simulink model "dog_x_bit_true_2024"  (R2024a)
settings: Solver=ode45  StartTime=0.0  StopTime=1.5*lsim*Ts  MaxStep=1/f0/2  RelTol=1e-6
values from neighbouring files (symbols this model uses):
  ft = (bint-1)*fbin    [exe_DOG_X_bit_true_2023a.m]    (also in exe_DOG_X_integer_true_two_paths_5b.m)
  g1 = g1_ideal*1    (= 4)    [exe_DOG_X_bit_true_2023a.m]    (also in exe_DOG_X_integer_true_two_paths_5b.m)
  Kvco = f0    (= 99840000)    [exe_DOG_X_bit_true_2023a.m]    (also in exe_DOG_X_integer_true_two_paths_5b.m)
  lvl = Vfs*10^(Input_signal_dB/20)    (= 0.125892541179)    [exe_DOG_X_bit_true_2023a.m]    (also in exe_DOG_X_integer_true_two_paths_5b.m)
  Nbsv1 = Nbvco+4    (= 9)    [exe_DOG_X_bit_true_2023a.m]    (also in exe_DOG_X_integer_true_two_paths_5b.m)
  Nbsv2 = Nbsv1+Nbext    [exe_DOG_X_bit_true_2023a.m]    (also in exe_DOG_X_integer_true_two_paths_5b.m)
  pnoi = 10^(-(60)/10)*(Vfs^2/2)    (= 5e-07)    [exe_DOG_X_bit_true_2023a.m]    (also in exe_DOG_X_integer_true_two_paths_5b.m)
  T2 = 1/f2    (= 4.06901041667e-08)    [exe_DOG_X_bit_true_2023a.m]    (also in exe_DOG_X_integer_true_two_paths_5b.m)
  Ts = 1/fs    (= 3.25520833333e-07)    [exe_DOG_X_bit_true_2023a.m]    (also in exe_DOG_X_integer_true_two_paths_5b.m)
  Vfs = 1    [exe_DOG_X_bit_true_2023a.m]    (also in exe_DOG_X_integer_true_two_paths_5b.m)
undefined symbols (not defined in the file or in its folder): fa, fb
libraries: simulink_extras x86, simulink x8
(part 3 of 4)

== system dog_x_bit_true_2024/TOP/Subsystem/progressive_mux/Subsystem1 ==
  select : Inport
  A : Inport  Port=2
  B : Inport  Port=3
  AND : Logic  IconShape=distinctive  AllPortsSameDT=off  OutDataTypeStr=boolean
  AND1 : Logic  IconShape=distinctive  AllPortsSameDT=off  OutDataTypeStr=boolean
  Demux : Demux  Outputs=15
  FA1 : Subsystem
  FA10 : Subsystem
  FA11 : Subsystem
  FA2 : Subsystem
  FA3 : Subsystem
  FA4 : Subsystem
  FA5 : Subsystem
  FA6 : Subsystem
  FA7 : Subsystem
  FA8 : Subsystem
  FA9 : Subsystem
  Mux : Mux
  NOT : Logic  Operator=NOT  IconShape=distinctive  AllPortsSameDT=off  OutDataTypeStr=boolean
  OR : Logic  Operator=OR  IconShape=distinctive  AllPortsSameDT=off  OutDataTypeStr=boolean
  Y : Outport
  wires:
  AND/1 -> OR/1
  A/1 -> AND/1
  AND1/1 -> OR/2
  B/1 -> AND1/2
  select/1 -> NOT/1, AND/2
  NOT/1 -> AND1/1
  OR/1 -> Demux/1
  Demux/2 -> FA10/3(Cin)
  Demux/15 -> FA10/1(B0)
  Demux/14 -> FA1/3(Cin)
  Demux/13 -> FA1/2(B1)
  Demux/12 -> FA1/1(B0)
  FA1/1(S) -> FA4/1(B0)
  FA10/1(S) -> FA4/2(B1)
  FA1/2(Co) -> FA5/2(B1)
  FA10/2(Co) -> FA5/1(B0)
  FA4/2(Co) -> FA5/3(Cin)
  Demux/11 -> FA4/3(Cin)
  FA6/2(Co) -> FA7/3(Cin)
  Demux/4 -> FA6/3(Cin)
  FA3/2(Co) -> FA7/1(B0)
  Demux/7 -> FA2/3(Cin)
  Demux/10 -> FA3/3(Cin)
  FA2/2(Co) -> FA7/2(B1)
  Demux/6 -> FA2/2(B1)
  Demux/9 -> FA3/2(B1)
  FA2/1(S) -> FA6/1(B0)
  FA3/1(S) -> FA6/2(B1)
  Demux/8 -> FA3/1(B0)
  Demux/5 -> FA2/1(B0)
  FA4/1(S) -> FA8/2(B1)
  FA5/1(S) -> FA9/2(B1)
  FA5/2(Co) -> FA11/2(B1)
  FA6/1(S) -> FA8/1(B0)
  FA7/1(S) -> FA9/1(B0)
  FA7/2(Co) -> FA11/1(B0)
  Demux/3 -> FA8/3(Cin)
  FA8/2(Co) -> FA9/3(Cin)
  FA9/2(Co) -> FA11/3(Cin)
  Demux/1 -> FA10/2(B1)
  FA11/2(Co) -> Mux/1
  FA11/1(S) -> Mux/2
  FA9/1(S) -> Mux/3
  FA8/1(S) -> Mux/4
  Mux/1 -> Y/1

== system dog_x_bit_true_2024/TOP/alpha2/abs/FA10 ==
  B0 : Inport
  B1 : Inport  Port=2
  Cin : Inport  Port=3
  Combinatorial Logic : CombinatorialLogic
  Demux : Demux  Outputs=2
  Mux : Mux  Inputs=3
  S : Outport
  Co : Outport  Port=2
  wires:
  Mux/1 -> Combinatorial Logic/1
  Combinatorial Logic/1 -> Demux/1
  B1/1 -> Mux/2
  Cin/1 -> Mux/3
  B0/1 -> Mux/1
  Demux/1 -> Co/1
  Demux/2 -> S/1

== system dog_x_bit_true_2024/TOP/alpha2/abs/FA2 ==
  B0 : Inport
  B1 : Inport  Port=2
  Cin : Inport  Port=3
  Combinatorial Logic : CombinatorialLogic
  Demux : Demux  Outputs=2
  Mux : Mux  Inputs=3
  S : Outport
  Co : Outport  Port=2
  wires:
  Mux/1 -> Combinatorial Logic/1
  Combinatorial Logic/1 -> Demux/1
  B1/1 -> Mux/2
  Cin/1 -> Mux/3
  B0/1 -> Mux/1
  Demux/1 -> Co/1
  Demux/2 -> S/1

== system dog_x_bit_true_2024/TOP/alpha2/abs/FA3 ==
  B0 : Inport
  B1 : Inport  Port=2
  Cin : Inport  Port=3
  Combinatorial Logic : CombinatorialLogic
  Demux : Demux  Outputs=2
  Mux : Mux  Inputs=3
  S : Outport
  Co : Outport  Port=2
  wires:
  Mux/1 -> Combinatorial Logic/1
  Combinatorial Logic/1 -> Demux/1
  B1/1 -> Mux/2
  Cin/1 -> Mux/3
  B0/1 -> Mux/1
  Demux/1 -> Co/1
  Demux/2 -> S/1

== system dog_x_bit_true_2024/TOP/alpha2/abs/FA4 ==
  B0 : Inport
  B1 : Inport  Port=2
  Cin : Inport  Port=3
  Combinatorial Logic : CombinatorialLogic
  Demux : Demux  Outputs=2
  Mux : Mux  Inputs=3
  S : Outport
  Co : Outport  Port=2
  wires:
  Mux/1 -> Combinatorial Logic/1
  Combinatorial Logic/1 -> Demux/1
  B1/1 -> Mux/2
  Cin/1 -> Mux/3
  B0/1 -> Mux/1
  Demux/1 -> Co/1
  Demux/2 -> S/1

== system dog_x_bit_true_2024/TOP/alpha2/abs/FA5 ==
  B0 : Inport
  B1 : Inport  Port=2
  Cin : Inport  Port=3
  Combinatorial Logic : CombinatorialLogic
  Demux : Demux  Outputs=2
  Mux : Mux  Inputs=3
  S : Outport
  Co : Outport  Port=2
  wires:
  Mux/1 -> Combinatorial Logic/1
  Combinatorial Logic/1 -> Demux/1
  B1/1 -> Mux/2
  Cin/1 -> Mux/3
  B0/1 -> Mux/1
  Demux/1 -> Co/1
  Demux/2 -> S/1

== system dog_x_bit_true_2024/TOP/alpha2/abs/FA6 ==
  B0 : Inport
  B1 : Inport  Port=2
  Cin : Inport  Port=3
  Combinatorial Logic : CombinatorialLogic
  Demux : Demux  Outputs=2
  Mux : Mux  Inputs=3
  S : Outport
  Co : Outport  Port=2
  wires:
  Mux/1 -> Combinatorial Logic/1
  Combinatorial Logic/1 -> Demux/1
  B1/1 -> Mux/2
  Cin/1 -> Mux/3
  B0/1 -> Mux/1
  Demux/1 -> Co/1
  Demux/2 -> S/1

== system dog_x_bit_true_2024/TOP/alpha2/abs/FA7 ==
  B0 : Inport
  B1 : Inport  Port=2
  Cin : Inport  Port=3
  Combinatorial Logic : CombinatorialLogic
  Demux : Demux  Outputs=2
  Mux : Mux  Inputs=3
  S : Outport
  Co : Outport  Port=2
  wires:
  Mux/1 -> Combinatorial Logic/1
  Combinatorial Logic/1 -> Demux/1
  B1/1 -> Mux/2
  Cin/1 -> Mux/3
  B0/1 -> Mux/1
  Demux/1 -> Co/1
  Demux/2 -> S/1

== system dog_x_bit_true_2024/TOP/alpha2/abs/FA9 ==
  B0 : Inport
  Cin : Inport  Port=2
  B1 : Inport  Port=3
  Combinatorial Logic : CombinatorialLogic
  Demux : Demux  Outputs=2
  Mux : Mux  Inputs=3
  S : Outport
  Co : Outport  Port=2
  wires:
  Mux/1 -> Combinatorial Logic/1
  Combinatorial Logic/1 -> Demux/1
  B1/1 -> Mux/2
  Cin/1 -> Mux/3
  B0/1 -> Mux/1
  Demux/1 -> Co/1
  Demux/2 -> S/1

== system dog_x_bit_true_2024/TOP/alpha2/comp_HI_Threshold/FA1 ==
  B0 : Inport
  B1 : Inport  Port=2
  Cin : Inport  Port=3
  Combinatorial Logic : CombinatorialLogic
  Demux : Demux  Outputs=2
  Mux : Mux  Inputs=3
  S : Outport
  Co : Outport  Port=2
  wires:
  Mux/1 -> Combinatorial Logic/1
  Combinatorial Logic/1 -> Demux/1
  B1/1 -> Mux/2
  Cin/1 -> Mux/3
  B0/1 -> Mux/1
  Demux/1 -> Co/1
  Demux/2 -> S/1

== system dog_x_bit_true_2024/TOP/alpha2/comp_HI_Threshold/FA10 ==
  B0 : Inport
  B1 : Inport  Port=2
  Cin : Inport  Port=3
  Combinatorial Logic : CombinatorialLogic
  Demux : Demux  Outputs=2
  Mux : Mux  Inputs=3
  S : Outport
  Co : Outport  Port=2
  wires:
  Mux/1 -> Combinatorial Logic/1
  Combinatorial Logic/1 -> Demux/1
  B1/1 -> Mux/2
  Cin/1 -> Mux/3
  B0/1 -> Mux/1
  Demux/1 -> Co/1
  Demux/2 -> S/1

== system dog_x_bit_true_2024/TOP/alpha2/comp_HI_Threshold/FA2 ==
  B0 : Inport
  B1 : Inport  Port=2
  Cin : Inport  Port=3
  Combinatorial Logic : CombinatorialLogic
  Demux : Demux  Outputs=2
  Mux : Mux  Inputs=3
  S : Outport
  Co : Outport  Port=2
  wires:
  Mux/1 -> Combinatorial Logic/1
  Combinatorial Logic/1 -> Demux/1
  B1/1 -> Mux/2
  Cin/1 -> Mux/3
  B0/1 -> Mux/1
  Demux/1 -> Co/1
  Demux/2 -> S/1

== system dog_x_bit_true_2024/TOP/alpha2/comp_HI_Threshold/FA3 ==
  B0 : Inport
  B1 : Inport  Port=2
  Cin : Inport  Port=3
  Combinatorial Logic : CombinatorialLogic
  Demux : Demux  Outputs=2
  Mux : Mux  Inputs=3
  S : Outport
  Co : Outport  Port=2
  wires:
  Mux/1 -> Combinatorial Logic/1
  Combinatorial Logic/1 -> Demux/1
  B1/1 -> Mux/2
  Cin/1 -> Mux/3
  B0/1 -> Mux/1
  Demux/1 -> Co/1
  Demux/2 -> S/1

== system dog_x_bit_true_2024/TOP/alpha2/comp_HI_Threshold/FA4 ==
  B0 : Inport
  B1 : Inport  Port=2
  Cin : Inport  Port=3
  Combinatorial Logic : CombinatorialLogic
  Demux : Demux  Outputs=2
  Mux : Mux  Inputs=3
  S : Outport
  Co : Outport  Port=2
  wires:
  Mux/1 -> Combinatorial Logic/1
  Combinatorial Logic/1 -> Demux/1
  B1/1 -> Mux/2
  Cin/1 -> Mux/3
  B0/1 -> Mux/1
  Demux/1 -> Co/1
  Demux/2 -> S/1

== system dog_x_bit_true_2024/TOP/alpha2/comp_HI_Threshold/FA5 ==
  B0 : Inport
  B1 : Inport  Port=2
  Cin : Inport  Port=3
  Combinatorial Logic : CombinatorialLogic
  Demux : Demux  Outputs=2
  Mux : Mux  Inputs=3
  S : Outport
  Co : Outport  Port=2
  wires:
  Mux/1 -> Combinatorial Logic/1
  Combinatorial Logic/1 -> Demux/1
  B1/1 -> Mux/2
  Cin/1 -> Mux/3
  B0/1 -> Mux/1
  Demux/1 -> Co/1
  Demux/2 -> S/1

== system dog_x_bit_true_2024/TOP/alpha2/comp_HI_Threshold/FA6 ==
  B0 : Inport
  B1 : Inport  Port=2
  Cin : Inport  Port=3
  Combinatorial Logic : CombinatorialLogic
  Demux : Demux  Outputs=2
  Mux : Mux  Inputs=3
  S : Outport
  Co : Outport  Port=2
  wires:
  Mux/1 -> Combinatorial Logic/1
  Combinatorial Logic/1 -> Demux/1
  B1/1 -> Mux/2
  Cin/1 -> Mux/3
  B0/1 -> Mux/1
  Demux/1 -> Co/1
  Demux/2 -> S/1

== system dog_x_bit_true_2024/TOP/alpha2/comp_HI_Threshold/FA7 ==
  B0 : Inport
  B1 : Inport  Port=2
  Cin : Inport  Port=3
  Combinatorial Logic : CombinatorialLogic
  Demux : Demux  Outputs=2
  Mux : Mux  Inputs=3
  S : Outport
  Co : Outport  Port=2
  wires:
  Mux/1 -> Combinatorial Logic/1
  Combinatorial Logic/1 -> Demux/1
  B1/1 -> Mux/2
  Cin/1 -> Mux/3
  B0/1 -> Mux/1
  Demux/1 -> Co/1
  Demux/2 -> S/1

== system dog_x_bit_true_2024/TOP/alpha2/comp_HI_Threshold/FA9 ==
  B0 : Inport
  Cin : Inport  Port=2
  B1 : Inport  Port=3
  Combinatorial Logic : CombinatorialLogic
  Demux : Demux  Outputs=2
  Mux : Mux  Inputs=3
  S : Outport
  Co : Outport  Port=2
  wires:
  Mux/1 -> Combinatorial Logic/1
  Combinatorial Logic/1 -> Demux/1
  B1/1 -> Mux/2
  Cin/1 -> Mux/3
  B0/1 -> Mux/1
  Demux/1 -> Co/1
  Demux/2 -> S/1

== system dog_x_bit_true_2024/TOP/alpha2/comp_LOW_Threshold/FA1 ==
  B0 : Inport
  B1 : Inport  Port=2
  Cin : Inport  Port=3
  Combinatorial Logic : CombinatorialLogic
  Demux : Demux  Outputs=2
  Mux : Mux  Inputs=3
  S : Outport
  Co : Outport  Port=2
  wires:
  Mux/1 -> Combinatorial Logic/1
  Combinatorial Logic/1 -> Demux/1
  B1/1 -> Mux/2
  Cin/1 -> Mux/3
  B0/1 -> Mux/1
  Demux/1 -> Co/1
  Demux/2 -> S/1

== system dog_x_bit_true_2024/TOP/alpha2/comp_LOW_Threshold/FA10 ==
  B0 : Inport
  B1 : Inport  Port=2
  Cin : Inport  Port=3
  Combinatorial Logic : CombinatorialLogic
  Demux : Demux  Outputs=2
  Mux : Mux  Inputs=3
  S : Outport
  Co : Outport  Port=2
  wires:
  Mux/1 -> Combinatorial Logic/1
  Combinatorial Logic/1 -> Demux/1
  B1/1 -> Mux/2
  Cin/1 -> Mux/3
  B0/1 -> Mux/1
  Demux/1 -> Co/1
  Demux/2 -> S/1

== system dog_x_bit_true_2024/TOP/alpha2/comp_LOW_Threshold/FA2 ==
  B0 : Inport
  B1 : Inport  Port=2
  Cin : Inport  Port=3
  Combinatorial Logic : CombinatorialLogic
  Demux : Demux  Outputs=2
  Mux : Mux  Inputs=3
  S : Outport
  Co : Outport  Port=2
  wires:
  Mux/1 -> Combinatorial Logic/1
  Combinatorial Logic/1 -> Demux/1
  B1/1 -> Mux/2
  Cin/1 -> Mux/3
  B0/1 -> Mux/1
  Demux/1 -> Co/1
  Demux/2 -> S/1

== system dog_x_bit_true_2024/TOP/alpha2/comp_LOW_Threshold/FA3 ==
  B0 : Inport
  B1 : Inport  Port=2
  Cin : Inport  Port=3
  Combinatorial Logic : CombinatorialLogic
  Demux : Demux  Outputs=2
  Mux : Mux  Inputs=3
  S : Outport
  Co : Outport  Port=2
  wires:
  Mux/1 -> Combinatorial Logic/1
  Combinatorial Logic/1 -> Demux/1
  B1/1 -> Mux/2
  Cin/1 -> Mux/3
  B0/1 -> Mux/1
  Demux/1 -> Co/1
  Demux/2 -> S/1

== system dog_x_bit_true_2024/TOP/alpha2/comp_LOW_Threshold/FA4 ==
  B0 : Inport
  B1 : Inport  Port=2
  Cin : Inport  Port=3
  Combinatorial Logic : CombinatorialLogic
  Demux : Demux  Outputs=2
  Mux : Mux  Inputs=3
  S : Outport
  Co : Outport  Port=2
  wires:
  Mux/1 -> Combinatorial Logic/1
  Combinatorial Logic/1 -> Demux/1
  B1/1 -> Mux/2
  Cin/1 -> Mux/3
  B0/1 -> Mux/1
  Demux/1 -> Co/1
  Demux/2 -> S/1

== system dog_x_bit_true_2024/TOP/alpha2/comp_LOW_Threshold/FA5 ==
  B0 : Inport
  B1 : Inport  Port=2
  Cin : Inport  Port=3
  Combinatorial Logic : CombinatorialLogic
  Demux : Demux  Outputs=2
  Mux : Mux  Inputs=3
  S : Outport
  Co : Outport  Port=2
  wires:
  Mux/1 -> Combinatorial Logic/1
  Combinatorial Logic/1 -> Demux/1
  B1/1 -> Mux/2
  Cin/1 -> Mux/3
  B0/1 -> Mux/1
  Demux/1 -> Co/1
  Demux/2 -> S/1

== system dog_x_bit_true_2024/TOP/alpha2/comp_LOW_Threshold/FA6 ==
  B0 : Inport
  B1 : Inport  Port=2
  Cin : Inport  Port=3
  Combinatorial Logic : CombinatorialLogic
  Demux : Demux  Outputs=2
  Mux : Mux  Inputs=3
  S : Outport
  Co : Outport  Port=2
  wires:
  Mux/1 -> Combinatorial Logic/1
  Combinatorial Logic/1 -> Demux/1
  B1/1 -> Mux/2
  Cin/1 -> Mux/3
  B0/1 -> Mux/1
  Demux/1 -> Co/1
  Demux/2 -> S/1

== system dog_x_bit_true_2024/TOP/alpha2/comp_LOW_Threshold/FA7 ==
  B0 : Inport
  B1 : Inport  Port=2
  Cin : Inport  Port=3
  Combinatorial Logic : CombinatorialLogic
  Demux : Demux  Outputs=2
  Mux : Mux  Inputs=3
  S : Outport
  Co : Outport  Port=2
  wires:
  Mux/1 -> Combinatorial Logic/1
  Combinatorial Logic/1 -> Demux/1
  B1/1 -> Mux/2
  Cin/1 -> Mux/3
  B0/1 -> Mux/1
  Demux/1 -> Co/1
  Demux/2 -> S/1

== system dog_x_bit_true_2024/TOP/alpha2/comp_LOW_Threshold/FA9 ==
  B0 : Inport
  Cin : Inport  Port=2
  B1 : Inport  Port=3
  Combinatorial Logic : CombinatorialLogic
  Demux : Demux  Outputs=2
  Mux : Mux  Inputs=3
  S : Outport
  Co : Outport  Port=2
  wires:
  Mux/1 -> Combinatorial Logic/1
  Combinatorial Logic/1 -> Demux/1
  B1/1 -> Mux/2
  Cin/1 -> Mux/3
  B0/1 -> Mux/1
  Demux/1 -> Co/1
  Demux/2 -> S/1

== system dog_x_bit_true_2024/TOP/Subsystem/Noise_shaper_HDR/DCO/accumulator (11 bits) ==
  plus : Inport
  feedback : Inport  Port=2
  Constant : Constant  Value=0  OutDataTypeStr=boolean
  Demux : Demux  Outputs=9
  Demux1 : Demux  Outputs=11
  FA1 : Subsystem
  FA11 : Subsystem
  FA12 : Subsystem
  FA13 : Subsystem
  FA2 : Subsystem
  FA3 : Subsystem
  FA4 : Subsystem
  FA5 : Subsystem
  FA6 : Subsystem
  FA7 : Subsystem
  FA8 : Subsystem
  Mux : Mux  Inputs=11
  Terminator : Terminator
  subs : Outport
  wires:
  FA1/2(Co) -> FA12/3(Cin)
  FA12/2(Co) -> FA11/3(Cin)
  FA4/2(Co) -> FA8/3(Cin)
  FA2/2(Co) -> FA1/3(Cin)
  FA8/2(Co) -> FA3/3(Cin)
  FA3/2(Co) -> FA2/3(Cin)
  FA5/2(Co) -> FA4/3(Cin)
  FA6/2(Co) -> FA5/3(Cin)
  FA7/2(Co) -> FA6/3(Cin)
  feedback/1 -> Demux1/1
  plus/1 -> Demux/1
  Mux/1 -> subs/1
  FA13/2(Co) -> FA7/3(Cin)
  Constant/1 -> FA13/3(Cin)
  Demux/9 -> FA13/2(B1)
  Demux/8 -> FA7/2(B1)
  Demux/7 -> FA6/2(B1)
  Demux/6 -> FA5/2(B1)
  Demux/5 -> FA4/2(B1)
  Demux/4 -> FA8/2(B1)
  Demux/3 -> FA3/2(B1)
  Demux/2 -> FA2/2(B1)
  Demux/1 -> FA11/2(B1), FA12/2(B1), FA1/2(B1)
  FA13/1(S) -> Mux/11
  FA7/1(S) -> Mux/10
  FA6/1(S) -> Mux/9
  FA5/1(S) -> Mux/8
  FA4/1(S) -> Mux/7
  FA8/1(S) -> Mux/6
  FA3/1(S) -> Mux/5
  FA2/1(S) -> Mux/4
  FA1/1(S) -> Mux/3
  FA12/1(S) -> Mux/2
  FA11/1(S) -> Mux/1
  FA11/2(Co) -> Terminator/1
  Demux1/1 -> FA11/1(B0)
  Demux1/2 -> FA12/1(B0)
  Demux1/3 -> FA1/1(B0)
  Demux1/4 -> FA2/1(B0)
  Demux1/5 -> FA3/1(B0)
  Demux1/6 -> FA8/1(B0)
  Demux1/7 -> FA4/1(B0)
  Demux1/8 -> FA5/1(B0)
  Demux1/9 -> FA6/1(B0)
  Demux1/10 -> FA7/1(B0)
  Demux1/11 -> FA13/1(B0)

== system dog_x_bit_true_2024/TOP/Subsystem/Noise_shaper_HDR/DCO/register1 ==
  CLK : Inport
  D : Inport  Port=2
  Constant4 : Constant  OutDataTypeStr=boolean
  D Flip-Flop : simulink_extras/Flip Flops/D Flip-Flop
  Terminator : Terminator
  Q : Outport
  wires:
  D/1 -> D Flip-Flop/1
  D Flip-Flop/1 -> Q/1
  D Flip-Flop/2 -> Terminator/1
  CLK/1 -> D Flip-Flop/2
  Constant4/1 -> D Flip-Flop/3

== system dog_x_bit_true_2024/TOP/Subsystem/Noise_shaper_HDR/differential substraction (9 bit)/FA ==
  B0 : Inport
  B1 : Inport  Port=2
  Cin : Inport  Port=3
  Combinatorial Logic : CombinatorialLogic
  Demux : Demux  Outputs=2
  Mux : Mux  Inputs=3
  S : Outport
  Co : Outport  Port=2
  wires:
  Mux/1 -> Combinatorial Logic/1
  Combinatorial Logic/1 -> Demux/1
  B1/1 -> Mux/2
  Cin/1 -> Mux/3
  B0/1 -> Mux/1
  Demux/1 -> Co/1
  Demux/2 -> S/1

== system dog_x_bit_true_2024/TOP/Subsystem/Noise_shaper_HDR/differential substraction (9 bit)/FA1 ==
  B0 : Inport
  B1 : Inport  Port=2
  Cin : Inport  Port=3
  Combinatorial Logic : CombinatorialLogic
  Demux : Demux  Outputs=2
  Mux : Mux  Inputs=3
  S : Outport
  Co : Outport  Port=2
  wires:
  Mux/1 -> Combinatorial Logic/1
  Combinatorial Logic/1 -> Demux/1
  B1/1 -> Mux/2
  Cin/1 -> Mux/3
  B0/1 -> Mux/1
  Demux/1 -> Co/1
  Demux/2 -> S/1

== system dog_x_bit_true_2024/TOP/Subsystem/Noise_shaper_HDR/differential substraction (9 bit)/FA2 ==
  B0 : Inport
  B1 : Inport  Port=2
  Cin : Inport  Port=3
  Combinatorial Logic : CombinatorialLogic
  Demux : Demux  Outputs=2
  Mux : Mux  Inputs=3
  S : Outport
  Co : Outport  Port=2
  wires:
  Mux/1 -> Combinatorial Logic/1
  Combinatorial Logic/1 -> Demux/1
  B1/1 -> Mux/2
  Cin/1 -> Mux/3
  B0/1 -> Mux/1
  Demux/1 -> Co/1
  Demux/2 -> S/1

== system dog_x_bit_true_2024/TOP/Subsystem/Noise_shaper_HDR/differential substraction (9 bit)/FA3 ==
  B0 : Inport
  B1 : Inport  Port=2
  Cin : Inport  Port=3
  Combinatorial Logic : CombinatorialLogic
  Demux : Demux  Outputs=2
  Mux : Mux  Inputs=3
  S : Outport
  Co : Outport  Port=2
  wires:
  Mux/1 -> Combinatorial Logic/1
  Combinatorial Logic/1 -> Demux/1
  B1/1 -> Mux/2
  Cin/1 -> Mux/3
  B0/1 -> Mux/1
  Demux/1 -> Co/1
  Demux/2 -> S/1

== system dog_x_bit_true_2024/TOP/Subsystem/Noise_shaper_HDR/differential substraction (9 bit)/FA4 ==
  B0 : Inport
  B1 : Inport  Port=2
  Cin : Inport  Port=3
  Combinatorial Logic : CombinatorialLogic
  Demux : Demux  Outputs=2
  Mux : Mux  Inputs=3
  S : Outport
  Co : Outport  Port=2
  wires:
  Mux/1 -> Combinatorial Logic/1
  Combinatorial Logic/1 -> Demux/1
  B1/1 -> Mux/2
  Cin/1 -> Mux/3
  B0/1 -> Mux/1
  Demux/1 -> Co/1
  Demux/2 -> S/1

== system dog_x_bit_true_2024/TOP/Subsystem/Noise_shaper_HDR/differential substraction (9 bit)/FA5 ==
  B0 : Inport
  B1 : Inport  Port=2
  Cin : Inport  Port=3
  Combinatorial Logic : CombinatorialLogic
  Demux : Demux  Outputs=2
  Mux : Mux  Inputs=3
  S : Outport
  Co : Outport  Port=2
  wires:
  Mux/1 -> Combinatorial Logic/1
  Combinatorial Logic/1 -> Demux/1
  B1/1 -> Mux/2
  Cin/1 -> Mux/3
  B0/1 -> Mux/1
  Demux/1 -> Co/1
  Demux/2 -> S/1

== system dog_x_bit_true_2024/TOP/Subsystem/Noise_shaper_HDR/differential substraction (9 bit)/FA6 ==
  B0 : Inport
  B1 : Inport  Port=2
  Cin : Inport  Port=3
  Combinatorial Logic : CombinatorialLogic
  Demux : Demux  Outputs=2
  Mux : Mux  Inputs=3
  S : Outport
  Co : Outport  Port=2
  wires:
  Mux/1 -> Combinatorial Logic/1
  Combinatorial Logic/1 -> Demux/1
  B1/1 -> Mux/2
  Cin/1 -> Mux/3
  B0/1 -> Mux/1
  Demux/1 -> Co/1
  Demux/2 -> S/1

== system dog_x_bit_true_2024/TOP/Subsystem/Noise_shaper_HDR/differential substraction (9 bit)/FA7 ==
  B0 : Inport
  B1 : Inport  Port=2
  Cin : Inport  Port=3
  Combinatorial Logic : CombinatorialLogic
  Demux : Demux  Outputs=2
  Mux : Mux  Inputs=3
  S : Outport
  Co : Outport  Port=2
  wires:
  Mux/1 -> Combinatorial Logic/1
  Combinatorial Logic/1 -> Demux/1
  B1/1 -> Mux/2
  Cin/1 -> Mux/3
  B0/1 -> Mux/1
  Demux/1 -> Co/1
  Demux/2 -> S/1

== system dog_x_bit_true_2024/TOP/Subsystem/Noise_shaper_HDR/differential substraction (9 bit)/FA8 ==
  B0 : Inport
  B1 : Inport  Port=2
  Cin : Inport  Port=3
  Combinatorial Logic : CombinatorialLogic
  Demux : Demux  Outputs=2
  Mux : Mux  Inputs=3
  S : Outport
  Co : Outport  Port=2
  wires:
  Mux/1 -> Combinatorial Logic/1
  Combinatorial Logic/1 -> Demux/1
  B1/1 -> Mux/2
  Cin/1 -> Mux/3
  B0/1 -> Mux/1
  Demux/1 -> Co/1
  Demux/2 -> S/1

== system dog_x_bit_true_2024/TOP/Subsystem/Noise_shaper_HDR/feedback substraction (9 bit)/FA ==
  B0 : Inport
  B1 : Inport  Port=2
  Cin : Inport  Port=3
  Combinatorial Logic : CombinatorialLogic
  Demux : Demux  Outputs=2
  Mux : Mux  Inputs=3
  S : Outport
  Co : Outport  Port=2
  wires:
  Mux/1 -> Combinatorial Logic/1
  Combinatorial Logic/1 -> Demux/1
  B1/1 -> Mux/2
  Cin/1 -> Mux/3
  B0/1 -> Mux/1
  Demux/1 -> Co/1
  Demux/2 -> S/1

== system dog_x_bit_true_2024/TOP/Subsystem/Noise_shaper_HDR/feedback substraction (9 bit)/FA1 ==
  B0 : Inport
  B1 : Inport  Port=2
  Cin : Inport  Port=3
  Combinatorial Logic : CombinatorialLogic
  Demux : Demux  Outputs=2
  Mux : Mux  Inputs=3
  S : Outport
  Co : Outport  Port=2
  wires:
  Mux/1 -> Combinatorial Logic/1
  Combinatorial Logic/1 -> Demux/1
  B1/1 -> Mux/2
  Cin/1 -> Mux/3
  B0/1 -> Mux/1
  Demux/1 -> Co/1
  Demux/2 -> S/1

== system dog_x_bit_true_2024/TOP/Subsystem/Noise_shaper_HDR/feedback substraction (9 bit)/FA2 ==
  B0 : Inport
  B1 : Inport  Port=2
  Cin : Inport  Port=3
  Combinatorial Logic : CombinatorialLogic
  Demux : Demux  Outputs=2
  Mux : Mux  Inputs=3
  S : Outport
  Co : Outport  Port=2
  wires:
  Mux/1 -> Combinatorial Logic/1
  Combinatorial Logic/1 -> Demux/1
  B1/1 -> Mux/2
  Cin/1 -> Mux/3
  B0/1 -> Mux/1
  Demux/1 -> Co/1
  Demux/2 -> S/1

== system dog_x_bit_true_2024/TOP/Subsystem/Noise_shaper_HDR/feedback substraction (9 bit)/FA3 ==
  B0 : Inport
  B1 : Inport  Port=2
  Cin : Inport  Port=3
  Combinatorial Logic : CombinatorialLogic
  Demux : Demux  Outputs=2
  Mux : Mux  Inputs=3
  S : Outport
  Co : Outport  Port=2
  wires:
  Mux/1 -> Combinatorial Logic/1
  Combinatorial Logic/1 -> Demux/1
  B1/1 -> Mux/2
  Cin/1 -> Mux/3
  B0/1 -> Mux/1
  Demux/1 -> Co/1
  Demux/2 -> S/1

== system dog_x_bit_true_2024/TOP/Subsystem/Noise_shaper_HDR/feedback substraction (9 bit)/FA4 ==
  B0 : Inport
  B1 : Inport  Port=2
  Cin : Inport  Port=3
  Combinatorial Logic : CombinatorialLogic
  Demux : Demux  Outputs=2
  Mux : Mux  Inputs=3
  S : Outport
  Co : Outport  Port=2
  wires:
  Mux/1 -> Combinatorial Logic/1
  Combinatorial Logic/1 -> Demux/1
  B1/1 -> Mux/2
  Cin/1 -> Mux/3
  B0/1 -> Mux/1
  Demux/1 -> Co/1
  Demux/2 -> S/1

== system dog_x_bit_true_2024/TOP/Subsystem/Noise_shaper_HDR/feedback substraction (9 bit)/FA5 ==
  B0 : Inport
  B1 : Inport  Port=2
  Cin : Inport  Port=3
  Combinatorial Logic : CombinatorialLogic
  Demux : Demux  Outputs=2
  Mux : Mux  Inputs=3
  S : Outport
  Co : Outport  Port=2
  wires:
  Mux/1 -> Combinatorial Logic/1
  Combinatorial Logic/1 -> Demux/1
  B1/1 -> Mux/2
  Cin/1 -> Mux/3
  B0/1 -> Mux/1
  Demux/1 -> Co/1
  Demux/2 -> S/1

== system dog_x_bit_true_2024/TOP/Subsystem/Noise_shaper_HDR/feedback substraction (9 bit)/FA6 ==
  B0 : Inport
  B1 : Inport  Port=2
  Cin : Inport  Port=3
  Combinatorial Logic : CombinatorialLogic
  Demux : Demux  Outputs=2
  Mux : Mux  Inputs=3
  S : Outport
  Co : Outport  Port=2
  wires:
  Mux/1 -> Combinatorial Logic/1
  Combinatorial Logic/1 -> Demux/1
  B1/1 -> Mux/2
  Cin/1 -> Mux/3
  B0/1 -> Mux/1
  Demux/1 -> Co/1
  Demux/2 -> S/1

== system dog_x_bit_true_2024/TOP/Subsystem/Noise_shaper_HDR/feedback substraction (9 bit)/FA7 ==
  B0 : Inport
  B1 : Inport  Port=2
  Cin : Inport  Port=3
  Combinatorial Logic : CombinatorialLogic
  Demux : Demux  Outputs=2
  Mux : Mux  Inputs=3
  S : Outport
  Co : Outport  Port=2
  wires:
  Mux/1 -> Combinatorial Logic/1
  Combinatorial Logic/1 -> Demux/1
  B1/1 -> Mux/2
  Cin/1 -> Mux/3
  B0/1 -> Mux/1
  Demux/1 -> Co/1
  Demux/2 -> S/1

== system dog_x_bit_true_2024/TOP/Subsystem/Noise_shaper_HDR/feedback substraction (9 bit)/FA8 ==
  B0 : Inport
  B1 : Inport  Port=2
  Cin : Inport  Port=3
  Combinatorial Logic : CombinatorialLogic
  Demux : Demux  Outputs=2
  Mux : Mux  Inputs=3
  S : Outport
  Co : Outport  Port=2
  wires:
  Mux/1 -> Combinatorial Logic/1
  Combinatorial Logic/1 -> Demux/1
  B1/1 -> Mux/2
  Cin/1 -> Mux/3
  B0/1 -> Mux/1
  Demux/1 -> Co/1
  Demux/2 -> S/1

== system dog_x_bit_true_2024/TOP/Subsystem/Noise_shaper_HDR/first difference substraction (9 bit)/FA ==
  B0 : Inport
  B1 : Inport  Port=2
  Cin : Inport  Port=3
  Combinatorial Logic : CombinatorialLogic
  Demux : Demux  Outputs=2
  Mux : Mux  Inputs=3
  S : Outport
  Co : Outport  Port=2
  wires:
  Mux/1 -> Combinatorial Logic/1
  Combinatorial Logic/1 -> Demux/1
  B1/1 -> Mux/2
  Cin/1 -> Mux/3
  B0/1 -> Mux/1
  Demux/1 -> Co/1
  Demux/2 -> S/1

== system dog_x_bit_true_2024/TOP/Subsystem/Noise_shaper_HDR/first difference substraction (9 bit)/FA1 ==
  B0 : Inport
  B1 : Inport  Port=2
  Cin : Inport  Port=3
  Combinatorial Logic : CombinatorialLogic
  Demux : Demux  Outputs=2
  Mux : Mux  Inputs=3
  S : Outport
  Co : Outport  Port=2
  wires:
  Mux/1 -> Combinatorial Logic/1
  Combinatorial Logic/1 -> Demux/1
  B1/1 -> Mux/2
  Cin/1 -> Mux/3
  B0/1 -> Mux/1
  Demux/1 -> Co/1
  Demux/2 -> S/1

== system dog_x_bit_true_2024/TOP/Subsystem/Noise_shaper_HDR/first difference substraction (9 bit)/FA2 ==
  B0 : Inport
  B1 : Inport  Port=2
  Cin : Inport  Port=3
  Combinatorial Logic : CombinatorialLogic
  Demux : Demux  Outputs=2
  Mux : Mux  Inputs=3
  S : Outport
  Co : Outport  Port=2
  wires:
  Mux/1 -> Combinatorial Logic/1
  Combinatorial Logic/1 -> Demux/1
  B1/1 -> Mux/2
  Cin/1 -> Mux/3
  B0/1 -> Mux/1
  Demux/1 -> Co/1
  Demux/2 -> S/1

== system dog_x_bit_true_2024/TOP/Subsystem/Noise_shaper_HDR/first difference substraction (9 bit)/FA3 ==
  B0 : Inport
  B1 : Inport  Port=2
  Cin : Inport  Port=3
  Combinatorial Logic : CombinatorialLogic
  Demux : Demux  Outputs=2
  Mux : Mux  Inputs=3
  S : Outport
  Co : Outport  Port=2
  wires:
  Mux/1 -> Combinatorial Logic/1
  Combinatorial Logic/1 -> Demux/1
  B1/1 -> Mux/2
  Cin/1 -> Mux/3
  B0/1 -> Mux/1
  Demux/1 -> Co/1
  Demux/2 -> S/1

== system dog_x_bit_true_2024/TOP/Subsystem/Noise_shaper_HDR/first difference substraction (9 bit)/FA4 ==
  B0 : Inport
  B1 : Inport  Port=2
  Cin : Inport  Port=3
  Combinatorial Logic : CombinatorialLogic
  Demux : Demux  Outputs=2
  Mux : Mux  Inputs=3
  S : Outport
  Co : Outport  Port=2
  wires:
  Mux/1 -> Combinatorial Logic/1
  Combinatorial Logic/1 -> Demux/1
  B1/1 -> Mux/2
  Cin/1 -> Mux/3
  B0/1 -> Mux/1
  Demux/1 -> Co/1
  Demux/2 -> S/1

== system dog_x_bit_true_2024/TOP/Subsystem/Noise_shaper_HDR/first difference substraction (9 bit)/FA5 ==
  B0 : Inport
  B1 : Inport  Port=2
  Cin : Inport  Port=3
  Combinatorial Logic : CombinatorialLogic
  Demux : Demux  Outputs=2
  Mux : Mux  Inputs=3
  S : Outport
  Co : Outport  Port=2
  wires:
  Mux/1 -> Combinatorial Logic/1
  Combinatorial Logic/1 -> Demux/1
  B1/1 -> Mux/2
  Cin/1 -> Mux/3
  B0/1 -> Mux/1
  Demux/1 -> Co/1
  Demux/2 -> S/1

== system dog_x_bit_true_2024/TOP/Subsystem/Noise_shaper_HDR/first difference substraction (9 bit)/FA6 ==
  B0 : Inport
  B1 : Inport  Port=2
  Cin : Inport  Port=3
  Combinatorial Logic : CombinatorialLogic
  Demux : Demux  Outputs=2
  Mux : Mux  Inputs=3
  S : Outport
  Co : Outport  Port=2
  wires:
  Mux/1 -> Combinatorial Logic/1
  Combinatorial Logic/1 -> Demux/1
  B1/1 -> Mux/2
  Cin/1 -> Mux/3
  B0/1 -> Mux/1
  Demux/1 -> Co/1
  Demux/2 -> S/1

== system dog_x_bit_true_2024/TOP/Subsystem/Noise_shaper_HDR/first difference substraction (9 bit)/FA7 ==
  B0 : Inport
  B1 : Inport  Port=2
  Cin : Inport  Port=3
  Combinatorial Logic : CombinatorialLogic
  Demux : Demux  Outputs=2
  Mux : Mux  Inputs=3
  S : Outport
  Co : Outport  Port=2
  wires:
  Mux/1 -> Combinatorial Logic/1
  Combinatorial Logic/1 -> Demux/1
  B1/1 -> Mux/2
  Cin/1 -> Mux/3
  B0/1 -> Mux/1
  Demux/1 -> Co/1
  Demux/2 -> S/1

== system dog_x_bit_true_2024/TOP/Subsystem/Noise_shaper_HDR/first difference substraction (9 bit)/FA8 ==
  B0 : Inport
  B1 : Inport  Port=2
  Cin : Inport  Port=3
  Combinatorial Logic : CombinatorialLogic
  Demux : Demux  Outputs=2
  Mux : Mux  Inputs=3
  S : Outport
  Co : Outport  Port=2
  wires:
  Mux/1 -> Combinatorial Logic/1
  Combinatorial Logic/1 -> Demux/1
  B1/1 -> Mux/2
  Cin/1 -> Mux/3
  B0/1 -> Mux/1
  Demux/1 -> Co/1
  Demux/2 -> S/1

== system dog_x_bit_true_2024/TOP/Subsystem/Noise_shaper_HDR/first difference substraction (9 bit)2/FA ==
  B0 : Inport
  B1 : Inport  Port=2
  Cin : Inport  Port=3
  Combinatorial Logic : CombinatorialLogic
  Demux : Demux  Outputs=2
  Mux : Mux  Inputs=3
  S : Outport
  Co : Outport  Port=2
  wires:
  Mux/1 -> Combinatorial Logic/1
  Combinatorial Logic/1 -> Demux/1
  B1/1 -> Mux/2
  Cin/1 -> Mux/3
  B0/1 -> Mux/1
  Demux/1 -> Co/1
  Demux/2 -> S/1

== system dog_x_bit_true_2024/TOP/Subsystem/Noise_shaper_HDR/first difference substraction (9 bit)2/FA1 ==
  B0 : Inport
  B1 : Inport  Port=2
  Cin : Inport  Port=3
  Combinatorial Logic : CombinatorialLogic
  Demux : Demux  Outputs=2
  Mux : Mux  Inputs=3
  S : Outport
  Co : Outport  Port=2
  wires:
  Mux/1 -> Combinatorial Logic/1
  Combinatorial Logic/1 -> Demux/1
  B1/1 -> Mux/2
  Cin/1 -> Mux/3
  B0/1 -> Mux/1
  Demux/1 -> Co/1
  Demux/2 -> S/1

== system dog_x_bit_true_2024/TOP/Subsystem/Noise_shaper_HDR/first difference substraction (9 bit)2/FA2 ==
  B0 : Inport
  B1 : Inport  Port=2
  Cin : Inport  Port=3
  Combinatorial Logic : CombinatorialLogic
  Demux : Demux  Outputs=2
  Mux : Mux  Inputs=3
  S : Outport
  Co : Outport  Port=2
  wires:
  Mux/1 -> Combinatorial Logic/1
  Combinatorial Logic/1 -> Demux/1
  B1/1 -> Mux/2
  Cin/1 -> Mux/3
  B0/1 -> Mux/1
  Demux/1 -> Co/1
  Demux/2 -> S/1

== system dog_x_bit_true_2024/TOP/Subsystem/Noise_shaper_HDR/first difference substraction (9 bit)2/FA3 ==
  B0 : Inport
  B1 : Inport  Port=2
  Cin : Inport  Port=3
  Combinatorial Logic : CombinatorialLogic
  Demux : Demux  Outputs=2
  Mux : Mux  Inputs=3
  S : Outport
  Co : Outport  Port=2
  wires:
  Mux/1 -> Combinatorial Logic/1
  Combinatorial Logic/1 -> Demux/1
  B1/1 -> Mux/2
  Cin/1 -> Mux/3
  B0/1 -> Mux/1
  Demux/1 -> Co/1
  Demux/2 -> S/1

== system dog_x_bit_true_2024/TOP/Subsystem/Noise_shaper_HDR/first difference substraction (9 bit)2/FA4 ==
  B0 : Inport
  B1 : Inport  Port=2
  Cin : Inport  Port=3
  Combinatorial Logic : CombinatorialLogic
  Demux : Demux  Outputs=2
  Mux : Mux  Inputs=3
  S : Outport
  Co : Outport  Port=2
  wires:
  Mux/1 -> Combinatorial Logic/1
  Combinatorial Logic/1 -> Demux/1
  B1/1 -> Mux/2
  Cin/1 -> Mux/3
  B0/1 -> Mux/1
  Demux/1 -> Co/1
  Demux/2 -> S/1

== system dog_x_bit_true_2024/TOP/Subsystem/Noise_shaper_HDR/first difference substraction (9 bit)2/FA5 ==
  B0 : Inport
  B1 : Inport  Port=2
  Cin : Inport  Port=3
  Combinatorial Logic : CombinatorialLogic
  Demux : Demux  Outputs=2
  Mux : Mux  Inputs=3
  S : Outport
  Co : Outport  Port=2
  wires:
  Mux/1 -> Combinatorial Logic/1
  Combinatorial Logic/1 -> Demux/1
  B1/1 -> Mux/2
  Cin/1 -> Mux/3
  B0/1 -> Mux/1
  Demux/1 -> Co/1
  Demux/2 -> S/1

== system dog_x_bit_true_2024/TOP/Subsystem/Noise_shaper_HDR/first difference substraction (9 bit)2/FA6 ==
  B0 : Inport
  B1 : Inport  Port=2
  Cin : Inport  Port=3
  Combinatorial Logic : CombinatorialLogic
  Demux : Demux  Outputs=2
  Mux : Mux  Inputs=3
  S : Outport
  Co : Outport  Port=2
  wires:
  Mux/1 -> Combinatorial Logic/1
  Combinatorial Logic/1 -> Demux/1
  B1/1 -> Mux/2
  Cin/1 -> Mux/3
  B0/1 -> Mux/1
  Demux/1 -> Co/1
  Demux/2 -> S/1

== system dog_x_bit_true_2024/TOP/Subsystem/Noise_shaper_HDR/first difference substraction (9 bit)2/FA7 ==
  B0 : Inport
  B1 : Inport  Port=2
  Cin : Inport  Port=3
  Combinatorial Logic : CombinatorialLogic
  Demux : Demux  Outputs=2
  Mux : Mux  Inputs=3
  S : Outport
  Co : Outport  Port=2
  wires:
  Mux/1 -> Combinatorial Logic/1
  Combinatorial Logic/1 -> Demux/1
  B1/1 -> Mux/2
  Cin/1 -> Mux/3
  B0/1 -> Mux/1
  Demux/1 -> Co/1
  Demux/2 -> S/1

== system dog_x_bit_true_2024/TOP/Subsystem/Noise_shaper_HDR/first difference substraction (9 bit)2/FA8 ==
  B0 : Inport
  B1 : Inport  Port=2
  Cin : Inport  Port=3
  Combinatorial Logic : CombinatorialLogic
  Demux : Demux  Outputs=2
  Mux : Mux  Inputs=3
  S : Outport
  Co : Outport  Port=2
  wires:
  Mux/1 -> Combinatorial Logic/1
  Combinatorial Logic/1 -> Demux/1
  B1/1 -> Mux/2
  Cin/1 -> Mux/3
  B0/1 -> Mux/1
  Demux/1 -> Co/1
  Demux/2 -> S/1

== system dog_x_bit_true_2024/TOP/Subsystem/Noise_shaper_HDR/offset correction/FA ==
  B0 : Inport
  B1 : Inport  Port=2
  Cin : Inport  Port=3
  Combinatorial Logic : CombinatorialLogic
  Demux : Demux  Outputs=2
  Mux : Mux  Inputs=3
  S : Outport
  Co : Outport  Port=2
  wires:
  Mux/1 -> Combinatorial Logic/1
  Combinatorial Logic/1 -> Demux/1
  B1/1 -> Mux/2
  Cin/1 -> Mux/3
  B0/1 -> Mux/1
  Demux/1 -> Co/1
  Demux/2 -> S/1

== system dog_x_bit_true_2024/TOP/Subsystem/Noise_shaper_HDR/offset correction/FA1 ==
  B0 : Inport
  B1 : Inport  Port=2
  Cin : Inport  Port=3
  Combinatorial Logic : CombinatorialLogic
  Demux : Demux  Outputs=2
  Mux : Mux  Inputs=3
  S : Outport
  Co : Outport  Port=2
  wires:
  Mux/1 -> Combinatorial Logic/1
  Combinatorial Logic/1 -> Demux/1
  B1/1 -> Mux/2
  Cin/1 -> Mux/3
  B0/1 -> Mux/1
  Demux/1 -> Co/1
  Demux/2 -> S/1

== system dog_x_bit_true_2024/TOP/Subsystem/Noise_shaper_HDR/offset correction/FA2 ==
  B0 : Inport
  B1 : Inport  Port=2
  Cin : Inport  Port=3
  Combinatorial Logic : CombinatorialLogic
  Demux : Demux  Outputs=2
  Mux : Mux  Inputs=3
  S : Outport
  Co : Outport  Port=2
  wires:
  Mux/1 -> Combinatorial Logic/1
  Combinatorial Logic/1 -> Demux/1
  B1/1 -> Mux/2
  Cin/1 -> Mux/3
  B0/1 -> Mux/1
  Demux/1 -> Co/1
  Demux/2 -> S/1

== system dog_x_bit_true_2024/TOP/Subsystem/Noise_shaper_HDR/offset correction/FA3 ==
  B0 : Inport
  B1 : Inport  Port=2
  Cin : Inport  Port=3
  Combinatorial Logic : CombinatorialLogic
  Demux : Demux  Outputs=2
  Mux : Mux  Inputs=3
  S : Outport
  Co : Outport  Port=2
  wires:
  Mux/1 -> Combinatorial Logic/1
  Combinatorial Logic/1 -> Demux/1
  B1/1 -> Mux/2
  Cin/1 -> Mux/3
  B0/1 -> Mux/1
  Demux/1 -> Co/1
  Demux/2 -> S/1

== system dog_x_bit_true_2024/TOP/Subsystem/Noise_shaper_HDR/offset correction/FA4 ==
  B0 : Inport
  B1 : Inport  Port=2
  Cin : Inport  Port=3
  Combinatorial Logic : CombinatorialLogic
  Demux : Demux  Outputs=2
  Mux : Mux  Inputs=3
  S : Outport
  Co : Outport  Port=2
  wires:
  Mux/1 -> Combinatorial Logic/1
  Combinatorial Logic/1 -> Demux/1
  B1/1 -> Mux/2
  Cin/1 -> Mux/3
  B0/1 -> Mux/1
  Demux/1 -> Co/1
  Demux/2 -> S/1

== system dog_x_bit_true_2024/TOP/Subsystem/Noise_shaper_HDR/offset correction/FA5 ==
  B0 : Inport
  B1 : Inport  Port=2
  Cin : Inport  Port=3
  Combinatorial Logic : CombinatorialLogic
  Demux : Demux  Outputs=2
  Mux : Mux  Inputs=3
  S : Outport
  Co : Outport  Port=2
  wires:
  Mux/1 -> Combinatorial Logic/1
  Combinatorial Logic/1 -> Demux/1
  B1/1 -> Mux/2
  Cin/1 -> Mux/3
  B0/1 -> Mux/1
  Demux/1 -> Co/1
  Demux/2 -> S/1

== system dog_x_bit_true_2024/TOP/Subsystem/Noise_shaper_HDR/offset correction/FA6 ==
  B0 : Inport
  B1 : Inport  Port=2
  Cin : Inport  Port=3
  Combinatorial Logic : CombinatorialLogic
  Demux : Demux  Outputs=2
  Mux : Mux  Inputs=3
  S : Outport
  Co : Outport  Port=2
  wires:
  Mux/1 -> Combinatorial Logic/1
  Combinatorial Logic/1 -> Demux/1
  B1/1 -> Mux/2
  Cin/1 -> Mux/3
  B0/1 -> Mux/1
  Demux/1 -> Co/1
  Demux/2 -> S/1

== system dog_x_bit_true_2024/TOP/Subsystem/Noise_shaper_HDR/offset correction/FA7 ==
  B0 : Inport
  B1 : Inport  Port=2
  Cin : Inport  Port=3
  Combinatorial Logic : CombinatorialLogic
  Demux : Demux  Outputs=2
  Mux : Mux  Inputs=3
  S : Outport
  Co : Outport  Port=2
  wires:
  Mux/1 -> Combinatorial Logic/1
  Combinatorial Logic/1 -> Demux/1
  B1/1 -> Mux/2
  Cin/1 -> Mux/3
  B0/1 -> Mux/1
  Demux/1 -> Co/1
  Demux/2 -> S/1

== system dog_x_bit_true_2024/TOP/Subsystem/Noise_shaper_HDR/offset correction/FA8 ==
  B0 : Inport
  B1 : Inport  Port=2
  Cin : Inport  Port=3
  Combinatorial Logic : CombinatorialLogic
  Demux : Demux  Outputs=2
  Mux : Mux  Inputs=3
  S : Outport
  Co : Outport  Port=2
  wires:
  Mux/1 -> Combinatorial Logic/1
  Combinatorial Logic/1 -> Demux/1
  B1/1 -> Mux/2
  Cin/1 -> Mux/3
  B0/1 -> Mux/1
  Demux/1 -> Co/1
  Demux/2 -> S/1

== system dog_x_bit_true_2024/TOP/Subsystem/Noise_shaper_HSNR/DCO/accumulator (11 bits) ==
  plus : Inport
  feedback : Inport  Port=2
  Constant : Constant  Value=0  OutDataTypeStr=boolean
  Demux : Demux  Outputs=9
  Demux1 : Demux  Outputs=11
  FA1 : Subsystem
  FA11 : Subsystem
  FA12 : Subsystem
  FA13 : Subsystem
  FA2 : Subsystem
  FA3 : Subsystem
  FA4 : Subsystem
  FA5 : Subsystem
  FA6 : Subsystem
  FA7 : Subsystem
  FA8 : Subsystem
  Mux : Mux  Inputs=11
  Terminator : Terminator
  subs : Outport
  wires:
  FA1/2(Co) -> FA12/3(Cin)
  FA12/2(Co) -> FA11/3(Cin)
  FA4/2(Co) -> FA8/3(Cin)
  FA2/2(Co) -> FA1/3(Cin)
  FA8/2(Co) -> FA3/3(Cin)
  FA3/2(Co) -> FA2/3(Cin)
  FA5/2(Co) -> FA4/3(Cin)
  FA6/2(Co) -> FA5/3(Cin)
  FA7/2(Co) -> FA6/3(Cin)
  feedback/1 -> Demux1/1
  plus/1 -> Demux/1
  Mux/1 -> subs/1
  FA13/2(Co) -> FA7/3(Cin)
  Constant/1 -> FA13/3(Cin)
  Demux/9 -> FA13/2(B1)
  Demux/8 -> FA7/2(B1)
  Demux/7 -> FA6/2(B1)
  Demux/6 -> FA5/2(B1)
  Demux/5 -> FA4/2(B1)
  Demux/4 -> FA8/2(B1)
  Demux/3 -> FA3/2(B1)
  Demux/2 -> FA2/2(B1)
  Demux/1 -> FA11/2(B1), FA12/2(B1), FA1/2(B1)
  FA13/1(S) -> Mux/11
  FA7/1(S) -> Mux/10
  FA6/1(S) -> Mux/9
  FA5/1(S) -> Mux/8
  FA4/1(S) -> Mux/7
  FA8/1(S) -> Mux/6
  FA3/1(S) -> Mux/5
  FA2/1(S) -> Mux/4
  FA1/1(S) -> Mux/3
  FA12/1(S) -> Mux/2
  FA11/1(S) -> Mux/1
  FA11/2(Co) -> Terminator/1
  Demux1/1 -> FA11/1(B0)
  Demux1/2 -> FA12/1(B0)
  Demux1/3 -> FA1/1(B0)
  Demux1/4 -> FA2/1(B0)
  Demux1/5 -> FA3/1(B0)
  Demux1/6 -> FA8/1(B0)
  Demux1/7 -> FA4/1(B0)
  Demux1/8 -> FA5/1(B0)
  Demux1/9 -> FA6/1(B0)
  Demux1/10 -> FA7/1(B0)
  Demux1/11 -> FA13/1(B0)

== system dog_x_bit_true_2024/TOP/Subsystem/Noise_shaper_HSNR/DCO/register1 ==
  CLK : Inport
  D : Inport  Port=2
  Constant4 : Constant  OutDataTypeStr=boolean
  D Flip-Flop : simulink_extras/Flip Flops/D Flip-Flop
  Terminator : Terminator
  Q : Outport
  wires:
  D/1 -> D Flip-Flop/1
  D Flip-Flop/1 -> Q/1
  D Flip-Flop/2 -> Terminator/1
  CLK/1 -> D Flip-Flop/2
  Constant4/1 -> D Flip-Flop/3

== system dog_x_bit_true_2024/TOP/Subsystem/Noise_shaper_HSNR/differential substraction (9 bit)/FA ==
  B0 : Inport
  B1 : Inport  Port=2
  Cin : Inport  Port=3
  Combinatorial Logic : CombinatorialLogic
  Demux : Demux  Outputs=2
  Mux : Mux  Inputs=3
  S : Outport
  Co : Outport  Port=2
  wires:
  Mux/1 -> Combinatorial Logic/1
  Combinatorial Logic/1 -> Demux/1
  B1/1 -> Mux/2
  Cin/1 -> Mux/3
  B0/1 -> Mux/1
  Demux/1 -> Co/1
  Demux/2 -> S/1

== system dog_x_bit_true_2024/TOP/Subsystem/Noise_shaper_HSNR/differential substraction (9 bit)/FA1 ==
  B0 : Inport
  B1 : Inport  Port=2
  Cin : Inport  Port=3
  Combinatorial Logic : CombinatorialLogic
  Demux : Demux  Outputs=2
  Mux : Mux  Inputs=3
  S : Outport
  Co : Outport  Port=2
  wires:
  Mux/1 -> Combinatorial Logic/1
  Combinatorial Logic/1 -> Demux/1
  B1/1 -> Mux/2
  Cin/1 -> Mux/3
  B0/1 -> Mux/1
  Demux/1 -> Co/1
  Demux/2 -> S/1

== system dog_x_bit_true_2024/TOP/Subsystem/Noise_shaper_HSNR/differential substraction (9 bit)/FA2 ==
  B0 : Inport
  B1 : Inport  Port=2
  Cin : Inport  Port=3
  Combinatorial Logic : CombinatorialLogic
  Demux : Demux  Outputs=2
  Mux : Mux  Inputs=3
  S : Outport
  Co : Outport  Port=2
  wires:
  Mux/1 -> Combinatorial Logic/1
  Combinatorial Logic/1 -> Demux/1
  B1/1 -> Mux/2
  Cin/1 -> Mux/3
  B0/1 -> Mux/1
  Demux/1 -> Co/1
  Demux/2 -> S/1

== system dog_x_bit_true_2024/TOP/Subsystem/Noise_shaper_HSNR/differential substraction (9 bit)/FA3 ==
  B0 : Inport
  B1 : Inport  Port=2
  Cin : Inport  Port=3
  Combinatorial Logic : CombinatorialLogic
  Demux : Demux  Outputs=2
  Mux : Mux  Inputs=3
  S : Outport
  Co : Outport  Port=2
  wires:
  Mux/1 -> Combinatorial Logic/1
  Combinatorial Logic/1 -> Demux/1
  B1/1 -> Mux/2
  Cin/1 -> Mux/3
  B0/1 -> Mux/1
  Demux/1 -> Co/1
  Demux/2 -> S/1

== system dog_x_bit_true_2024/TOP/Subsystem/Noise_shaper_HSNR/differential substraction (9 bit)/FA4 ==
  B0 : Inport
  B1 : Inport  Port=2
  Cin : Inport  Port=3
  Combinatorial Logic : CombinatorialLogic
  Demux : Demux  Outputs=2
  Mux : Mux  Inputs=3
  S : Outport
  Co : Outport  Port=2
  wires:
  Mux/1 -> Combinatorial Logic/1
  Combinatorial Logic/1 -> Demux/1
  B1/1 -> Mux/2
  Cin/1 -> Mux/3
  B0/1 -> Mux/1
  Demux/1 -> Co/1
  Demux/2 -> S/1

== system dog_x_bit_true_2024/TOP/Subsystem/Noise_shaper_HSNR/differential substraction (9 bit)/FA5 ==
  B0 : Inport
  B1 : Inport  Port=2
  Cin : Inport  Port=3
  Combinatorial Logic : CombinatorialLogic
  Demux : Demux  Outputs=2
  Mux : Mux  Inputs=3
  S : Outport
  Co : Outport  Port=2
  wires:
  Mux/1 -> Combinatorial Logic/1
  Combinatorial Logic/1 -> Demux/1
  B1/1 -> Mux/2
  Cin/1 -> Mux/3
  B0/1 -> Mux/1
  Demux/1 -> Co/1
  Demux/2 -> S/1

== system dog_x_bit_true_2024/TOP/Subsystem/Noise_shaper_HSNR/differential substraction (9 bit)/FA6 ==
  B0 : Inport
  B1 : Inport  Port=2
  Cin : Inport  Port=3
  Combinatorial Logic : CombinatorialLogic
  Demux : Demux  Outputs=2
  Mux : Mux  Inputs=3
  S : Outport
  Co : Outport  Port=2
  wires:
  Mux/1 -> Combinatorial Logic/1
  Combinatorial Logic/1 -> Demux/1
  B1/1 -> Mux/2
  Cin/1 -> Mux/3
  B0/1 -> Mux/1
  Demux/1 -> Co/1
  Demux/2 -> S/1

== system dog_x_bit_true_2024/TOP/Subsystem/Noise_shaper_HSNR/differential substraction (9 bit)/FA7 ==
  B0 : Inport
  B1 : Inport  Port=2
  Cin : Inport  Port=3
  Combinatorial Logic : CombinatorialLogic
  Demux : Demux  Outputs=2
  Mux : Mux  Inputs=3
  S : Outport
  Co : Outport  Port=2
  wires:
  Mux/1 -> Combinatorial Logic/1
  Combinatorial Logic/1 -> Demux/1
  B1/1 -> Mux/2
  Cin/1 -> Mux/3
  B0/1 -> Mux/1
  Demux/1 -> Co/1
  Demux/2 -> S/1

== system dog_x_bit_true_2024/TOP/Subsystem/Noise_shaper_HSNR/differential substraction (9 bit)/FA8 ==
  B0 : Inport
  B1 : Inport  Port=2
  Cin : Inport  Port=3
  Combinatorial Logic : CombinatorialLogic
  Demux : Demux  Outputs=2
  Mux : Mux  Inputs=3
  S : Outport
  Co : Outport  Port=2
  wires:
  Mux/1 -> Combinatorial Logic/1
  Combinatorial Logic/1 -> Demux/1
  B1/1 -> Mux/2
  Cin/1 -> Mux/3
  B0/1 -> Mux/1
  Demux/1 -> Co/1
  Demux/2 -> S/1

== system dog_x_bit_true_2024/TOP/Subsystem/Noise_shaper_HSNR/feedback substraction (9 bit)/FA ==
  B0 : Inport
  B1 : Inport  Port=2
  Cin : Inport  Port=3
  Combinatorial Logic : CombinatorialLogic
  Demux : Demux  Outputs=2
  Mux : Mux  Inputs=3
  S : Outport
  Co : Outport  Port=2
  wires:
  Mux/1 -> Combinatorial Logic/1
  Combinatorial Logic/1 -> Demux/1
  B1/1 -> Mux/2
  Cin/1 -> Mux/3
  B0/1 -> Mux/1
  Demux/1 -> Co/1
  Demux/2 -> S/1

== system dog_x_bit_true_2024/TOP/Subsystem/Noise_shaper_HSNR/feedback substraction (9 bit)/FA1 ==
  B0 : Inport
  B1 : Inport  Port=2
  Cin : Inport  Port=3
  Combinatorial Logic : CombinatorialLogic
  Demux : Demux  Outputs=2
  Mux : Mux  Inputs=3
  S : Outport
  Co : Outport  Port=2
  wires:
  Mux/1 -> Combinatorial Logic/1
  Combinatorial Logic/1 -> Demux/1
  B1/1 -> Mux/2
  Cin/1 -> Mux/3
  B0/1 -> Mux/1
  Demux/1 -> Co/1
  Demux/2 -> S/1

== system dog_x_bit_true_2024/TOP/Subsystem/Noise_shaper_HSNR/feedback substraction (9 bit)/FA2 ==
  B0 : Inport
  B1 : Inport  Port=2
  Cin : Inport  Port=3
  Combinatorial Logic : CombinatorialLogic
  Demux : Demux  Outputs=2
  Mux : Mux  Inputs=3
  S : Outport
  Co : Outport  Port=2
  wires:
  Mux/1 -> Combinatorial Logic/1
  Combinatorial Logic/1 -> Demux/1
  B1/1 -> Mux/2
  Cin/1 -> Mux/3
  B0/1 -> Mux/1
  Demux/1 -> Co/1
  Demux/2 -> S/1

== system dog_x_bit_true_2024/TOP/Subsystem/Noise_shaper_HSNR/feedback substraction (9 bit)/FA3 ==
  B0 : Inport
  B1 : Inport  Port=2
  Cin : Inport  Port=3
  Combinatorial Logic : CombinatorialLogic
  Demux : Demux  Outputs=2
  Mux : Mux  Inputs=3
  S : Outport
  Co : Outport  Port=2
  wires:
  Mux/1 -> Combinatorial Logic/1
  Combinatorial Logic/1 -> Demux/1
  B1/1 -> Mux/2
  Cin/1 -> Mux/3
  B0/1 -> Mux/1
  Demux/1 -> Co/1
  Demux/2 -> S/1

== system dog_x_bit_true_2024/TOP/Subsystem/Noise_shaper_HSNR/feedback substraction (9 bit)/FA4 ==
  B0 : Inport
  B1 : Inport  Port=2
  Cin : Inport  Port=3
  Combinatorial Logic : CombinatorialLogic
  Demux : Demux  Outputs=2
  Mux : Mux  Inputs=3
  S : Outport
  Co : Outport  Port=2
  wires:
  Mux/1 -> Combinatorial Logic/1
  Combinatorial Logic/1 -> Demux/1
  B1/1 -> Mux/2
  Cin/1 -> Mux/3
  B0/1 -> Mux/1
  Demux/1 -> Co/1
  Demux/2 -> S/1

== system dog_x_bit_true_2024/TOP/Subsystem/Noise_shaper_HSNR/feedback substraction (9 bit)/FA5 ==
  B0 : Inport
  B1 : Inport  Port=2
  Cin : Inport  Port=3
  Combinatorial Logic : CombinatorialLogic
  Demux : Demux  Outputs=2
  Mux : Mux  Inputs=3
  S : Outport
  Co : Outport  Port=2
  wires:
  Mux/1 -> Combinatorial Logic/1
  Combinatorial Logic/1 -> Demux/1
  B1/1 -> Mux/2
  Cin/1 -> Mux/3
  B0/1 -> Mux/1
  Demux/1 -> Co/1
  Demux/2 -> S/1

== system dog_x_bit_true_2024/TOP/Subsystem/Noise_shaper_HSNR/feedback substraction (9 bit)/FA6 ==
  B0 : Inport
  B1 : Inport  Port=2
  Cin : Inport  Port=3
  Combinatorial Logic : CombinatorialLogic
  Demux : Demux  Outputs=2
  Mux : Mux  Inputs=3
  S : Outport
  Co : Outport  Port=2
  wires:
  Mux/1 -> Combinatorial Logic/1
  Combinatorial Logic/1 -> Demux/1
  B1/1 -> Mux/2
  Cin/1 -> Mux/3
  B0/1 -> Mux/1
  Demux/1 -> Co/1
  Demux/2 -> S/1

== system dog_x_bit_true_2024/TOP/Subsystem/Noise_shaper_HSNR/feedback substraction (9 bit)/FA7 ==
  B0 : Inport
  B1 : Inport  Port=2
  Cin : Inport  Port=3
  Combinatorial Logic : CombinatorialLogic
  Demux : Demux  Outputs=2
  Mux : Mux  Inputs=3
  S : Outport
  Co : Outport  Port=2
  wires:
  Mux/1 -> Combinatorial Logic/1
  Combinatorial Logic/1 -> Demux/1
  B1/1 -> Mux/2
  Cin/1 -> Mux/3
  B0/1 -> Mux/1
  Demux/1 -> Co/1
  Demux/2 -> S/1

== system dog_x_bit_true_2024/TOP/Subsystem/Noise_shaper_HSNR/feedback substraction (9 bit)/FA8 ==
  B0 : Inport
  B1 : Inport  Port=2
  Cin : Inport  Port=3
  Combinatorial Logic : CombinatorialLogic
  Demux : Demux  Outputs=2
  Mux : Mux  Inputs=3
  S : Outport
  Co : Outport  Port=2
  wires:
  Mux/1 -> Combinatorial Logic/1
  Combinatorial Logic/1 -> Demux/1
  B1/1 -> Mux/2
  Cin/1 -> Mux/3
  B0/1 -> Mux/1
  Demux/1 -> Co/1
  Demux/2 -> S/1

== system dog_x_bit_true_2024/TOP/Subsystem/Noise_shaper_HSNR/first difference substraction (9 bit)/FA ==
  B0 : Inport
  B1 : Inport  Port=2
  Cin : Inport  Port=3
  Combinatorial Logic : CombinatorialLogic
  Demux : Demux  Outputs=2
  Mux : Mux  Inputs=3
  S : Outport
  Co : Outport  Port=2
  wires:
  Mux/1 -> Combinatorial Logic/1
  Combinatorial Logic/1 -> Demux/1
  B1/1 -> Mux/2
  Cin/1 -> Mux/3
  B0/1 -> Mux/1
  Demux/1 -> Co/1
  Demux/2 -> S/1

== system dog_x_bit_true_2024/TOP/Subsystem/Noise_shaper_HSNR/first difference substraction (9 bit)/FA1 ==
  B0 : Inport
  B1 : Inport  Port=2
  Cin : Inport  Port=3
  Combinatorial Logic : CombinatorialLogic
  Demux : Demux  Outputs=2
  Mux : Mux  Inputs=3
  S : Outport
  Co : Outport  Port=2
  wires:
  Mux/1 -> Combinatorial Logic/1
  Combinatorial Logic/1 -> Demux/1
  B1/1 -> Mux/2
  Cin/1 -> Mux/3
  B0/1 -> Mux/1
  Demux/1 -> Co/1
  Demux/2 -> S/1

== system dog_x_bit_true_2024/TOP/Subsystem/Noise_shaper_HSNR/first difference substraction (9 bit)/FA2 ==
  B0 : Inport
  B1 : Inport  Port=2
  Cin : Inport  Port=3
  Combinatorial Logic : CombinatorialLogic
  Demux : Demux  Outputs=2
  Mux : Mux  Inputs=3
  S : Outport
  Co : Outport  Port=2
  wires:
  Mux/1 -> Combinatorial Logic/1
  Combinatorial Logic/1 -> Demux/1
  B1/1 -> Mux/2
  Cin/1 -> Mux/3
  B0/1 -> Mux/1
  Demux/1 -> Co/1
  Demux/2 -> S/1

== system dog_x_bit_true_2024/TOP/Subsystem/Noise_shaper_HSNR/first difference substraction (9 bit)/FA3 ==
  B0 : Inport
  B1 : Inport  Port=2
  Cin : Inport  Port=3
  Combinatorial Logic : CombinatorialLogic
  Demux : Demux  Outputs=2
  Mux : Mux  Inputs=3
  S : Outport
  Co : Outport  Port=2
  wires:
  Mux/1 -> Combinatorial Logic/1
  Combinatorial Logic/1 -> Demux/1
  B1/1 -> Mux/2
  Cin/1 -> Mux/3
  B0/1 -> Mux/1
  Demux/1 -> Co/1
  Demux/2 -> S/1

== system dog_x_bit_true_2024/TOP/Subsystem/Noise_shaper_HSNR/first difference substraction (9 bit)/FA4 ==
  B0 : Inport
  B1 : Inport  Port=2
  Cin : Inport  Port=3
  Combinatorial Logic : CombinatorialLogic
  Demux : Demux  Outputs=2
  Mux : Mux  Inputs=3
  S : Outport
  Co : Outport  Port=2
  wires:
  Mux/1 -> Combinatorial Logic/1
  Combinatorial Logic/1 -> Demux/1
  B1/1 -> Mux/2
  Cin/1 -> Mux/3
  B0/1 -> Mux/1
  Demux/1 -> Co/1
  Demux/2 -> S/1

== system dog_x_bit_true_2024/TOP/Subsystem/Noise_shaper_HSNR/first difference substraction (9 bit)/FA5 ==
  B0 : Inport
  B1 : Inport  Port=2
  Cin : Inport  Port=3
  Combinatorial Logic : CombinatorialLogic
  Demux : Demux  Outputs=2
  Mux : Mux  Inputs=3
  S : Outport
  Co : Outport  Port=2
  wires:
  Mux/1 -> Combinatorial Logic/1
  Combinatorial Logic/1 -> Demux/1
  B1/1 -> Mux/2
  Cin/1 -> Mux/3
  B0/1 -> Mux/1
  Demux/1 -> Co/1
  Demux/2 -> S/1

== system dog_x_bit_true_2024/TOP/Subsystem/Noise_shaper_HSNR/first difference substraction (9 bit)/FA6 ==
  B0 : Inport
  B1 : Inport  Port=2
  Cin : Inport  Port=3
  Combinatorial Logic : CombinatorialLogic
  Demux : Demux  Outputs=2
  Mux : Mux  Inputs=3
  S : Outport
  Co : Outport  Port=2
  wires:
  Mux/1 -> Combinatorial Logic/1
  Combinatorial Logic/1 -> Demux/1
  B1/1 -> Mux/2
  Cin/1 -> Mux/3
  B0/1 -> Mux/1
  Demux/1 -> Co/1
  Demux/2 -> S/1
